simulink model "SimulacionOchoEstados"  (R2022b)
settings: Solver=VariableStepAuto  StartTime=0.0  StopTime=60  RelTol=1e-3
undefined symbols (not defined in the file): A, B, k1, k2, nodos, P, W1_0, W2_0
settings Model: Creator=raul  LastModifiedBy=raul

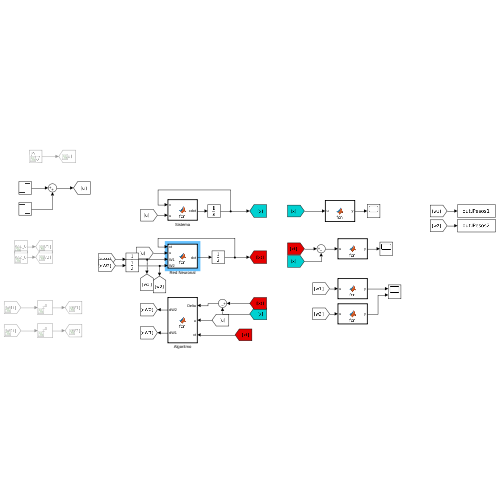
[thumbnail: Simulink's stored preview of the top-level diagram]
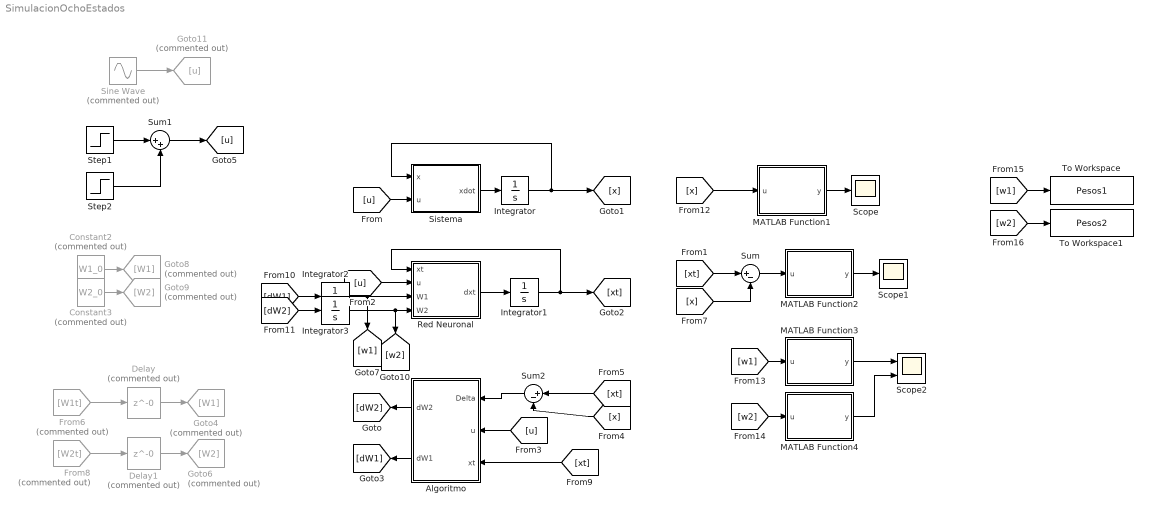
== system SimulacionOchoEstados ==
  Algoritmo : MATLAB Function  TreatAsAtomicUnit=on
  Constant2 : Constant  Commented=on  Value=W1_0
  Constant3 : Constant  Commented=on  Value=W2_0
  Delay : Delay  Commented=on  DelayLength=0  InitialCondition=W1_0
  Delay1 : Delay  Commented=on  DelayLength=0  InitialCondition=W2_0
  From6 : From  Commented=on  GotoTag=W1t
  From8 : From  Commented=on  GotoTag=W2t
  Goto11 : Goto  Commented=on  GotoTag=u
  Goto4 : Goto  Commented=on  GotoTag=W1
  Goto6 : Goto  Commented=on  GotoTag=W2
  Goto8 : Goto  Commented=on  GotoTag=W1
  Goto9 : Goto  Commented=on  GotoTag=W2
  Integrator : Integrator  InitialCondition=zeros(2*nodos,nodos)
  Integrator1 : Integrator  InitialCondition=zeros(2*nodos,nodos)
  Integrator2 : Integrator  InitialCondition=W1_0
  Integrator3 : Integrator  InitialCondition=W2_0
  MATLAB Function1 : MATLAB Function  TreatAsAtomicUnit=on
  MATLAB Function2 : MATLAB Function  TreatAsAtomicUnit=on
  MATLAB Function3 : MATLAB Function  TreatAsAtomicUnit=on
  MATLAB Function4 : MATLAB Function  TreatAsAtomicUnit=on
  Red Neuronal : MATLAB Function  TreatAsAtomicUnit=on
  Scope : Scope
  Scope1 : Scope
  Scope2 : Scope  NumInputPorts=2
  Sine Wave : Sin  Commented=on  SampleTime=0
  Sistema : MATLAB Function  TreatAsAtomicUnit=on
  Step1 : Step  SampleTime=0
  Step2 : Step  Time=1.1  After=-1  SampleTime=0
  Sum : Sum  Inputs=|+-
  Sum1 : Sum  Inputs=|++
  Sum2 : Sum  Inputs=|+-
  To Workspace : ToWorkspace  VariableName=Pesos1  SampleTime=-1
  To Workspace1 : ToWorkspace  VariableName=Pesos2  SampleTime=-1
  wires:
  Sistema/1(xdot) -> Integrator/1
  Integrator/1 -> [x], Sistema/1(x)
  Step1/1 -> Sum1/1
  Sum1/1 -> [u]
  Step2/1 -> Sum1/2
  [u] -> Sistema/2(u)
  Integrator1/1 -> [xt], Red Neuronal/1(xt)
  [u] -> Red Neuronal/2(u)
  Red Neuronal/1(dxt) -> Integrator1/1
  Constant2/1 -> Goto8/1
  Constant3/1 -> Goto9/1
  [xt] -> Sum2/1
  Sum2/1 -> Algoritmo/1(Delta)
  [u] -> Algoritmo/2(u)
  [x] -> Sum2/2
  [xt] -> Algoritmo/3(xt)
  MATLAB Function1/1(y) -> Scope/1
  [x] -> MATLAB Function1/1(u)
  Sum/1 -> MATLAB Function2/1(u)
  MATLAB Function2/1(y) -> Scope1/1
  [xt] -> Sum/1
  [x] -> Sum/2
  From6/1 -> Delay/1
  From8/1 -> Delay1/1
  Delay/1 -> Goto4/1
  Delay1/1 -> Goto6/1
  Algoritmo/1(dW2) -> [dW2]
  Algoritmo/2(dW1) -> [dW1]
  Integrator3/1 -> [w2], Red Neuronal/4(W2)
  [dW1] -> Integrator2/1
  [dW2] -> Integrator3/1
  Integrator2/1 -> [w1], Red Neuronal/3(W1)
  [w1] -> MATLAB Function3/1(u)
  [w2] -> MATLAB Function4/1(u)
  MATLAB Function3/1(y) -> Scope2/1
  MATLAB Function4/1(y) -> Scope2/2
  [w1] -> To Workspace/1
  [w2] -> To Workspace1/1
  Sine Wave/1 -> Goto11/1

== matlab function SimulacionOchoEstados/Red Neuronal ==
  data: xt input; u input; dxt output; W1 input; A parameter; W2 input
function dxt = fcn(xt, u, W1, A, W2)

dxt = A*xt+W1*sigmoid(1,xt)+W2*sigmoid(1,xt)*u;


function s = sigmoid(b,x)
   s = 1./(1+exp(-b*x)); 
end

end

== matlab function SimulacionOchoEstados/Sistema ==
  data: x input; u input; xdot output; A parameter; B parameter
function xdot = fcn(x,u,A, B)

xdot = A*x+B*u;

== matlab function SimulacionOchoEstados/Algoritmo ==
  data: dW2 output; Delta input; P parameter; u input; dW1 output; k1 parameter; k2 parameter; xt input
function [dW2,dW1] = fcn(Delta,P,u, k1, k2,xt)


dW1=-k1*P*Delta*sigmoid(1,xt)';
dW2=-k2*P*Delta*sigmoid(1,xt)'*u;

function s = sigmoid(b,x)
   s = 1./(1+exp(-b*x)); 
end

end

== matlab function SimulacionOchoEstados/MATLAB Function2 ==
  data: u input; y output; f parameter
function y = fcn(u,f)

y = u(:,f);

== matlab function SimulacionOchoEstados/MATLAB Function1 ==
  data: u input; y output; f parameter
function y = fcn(u,f)

y = u(:,f);

== matlab function SimulacionOchoEstados/MATLAB Function3 ==
  data: u input; y output; f parameter
function y = fcn(u,f)

y = u(:,f);

== matlab function SimulacionOchoEstados/MATLAB Function4 ==
  data: u input; y output; f parameter
function y = fcn(u,f)

y = u(:,f);
